simulink model "TrajectoryControl_Team"  (R2022b)
settings: Solver=FixedStepAuto  StartTime=0.0  StopTime=30  FixedStep=0.001  RelTol=1e-3
undefined symbols (not defined in the file): h, headingAngle, km, m, Moment_limit, s, smiData, Steering_Angle, Vehicle_Speed, x, X, Y, Z
libraries: sm_lib x213, aerolibconvert2 x17, simulink_extras x14, nesl_utility x14, spsMosfetLib x4, autolibshared x3, slpidlib x2, eePwmGenerator x1, spsDCVoltageSourceLib x1, spsVoltageMeasurementLib x1, sps_lib x1, autolibutils x1
(part 1 of 6)
settings Model: Creator=dangm  LastModifiedBy=Lenovo
settings SolverCC: ZeroCrossAlgorithm=Adaptive  AlgebraicLoopSolver=LineSearch
settings DebuggingCC: IgnoredZcDiagnostic=none  UnconnectedInputMsg=warning  UnconnectedOutputMsg=warning  UnconnectedLineMsg=warning  SFMachineParentedDataDiag=warning
settings ModelReferenceCC: EnableRefExpFcnMdlSchedulingChecks=on
settings ExplorerConfigSet: InternalSimMechanicsExplorerSettings="<ExplorerConfiguration><canonicalview>planar_xy</canonicalview><AnimationSetting><BasePlaybackSpeed>1.0</BasePlaybackSpeed><PlaybackSpeedFactor>1.0</PlaybackSpeedFactor></AnimationSetting><TilePanel><TileInfo><Tiles Columns=\"1\" Count=\"1\" Rows=\"1\"><Column Weight=\"1\"/><Row Weight=\"1\"/><Tile Height=\"1\" Width=\"1\" X=\"0\" Y=\"0\"/></Tiles></TileInfo><SceneInfo><SceneViewer><BGColor><R>0.60000002384185791</R><G>0.60000002384185791</G><B>0.60000002384185791</B></BGColor><Camera><DoPerspective>off</DoPerspective><Position><X>1.38151927744802361</X><Y>-0.113937833645223696</Y><Z>-0.183681847979671575</Z></Position><Center><X>0.0576620377884289326</X><Y>0.060665039066758325</Y><Z>0.733764197719871003</Z></Center><Up><X>0.27535581417737931</X><Y>0.936019488942585909</Y><Z>0.219195556338108416</Z></Up><ViewLimDist>1</ViewLimDist><YLim>0.747285369634628327</YLim><XLim>1.35610315607225207</XLim></Camera></SceneViewer></SceneInfo></TilePanel><MechEditorPanel><Cameras/><GfxPanelCameraMap/><VideoCreator><PlaybackSpeedRatio>1.0</PlaybackSpeedRatio><FrameRate>30</FrameRate><VideoFormat>Motion JPEG AVI</VideoFormat><FrameSize>auto</FrameSize></VideoCreator></MechEditorPanel></ExplorerConfiguration>"

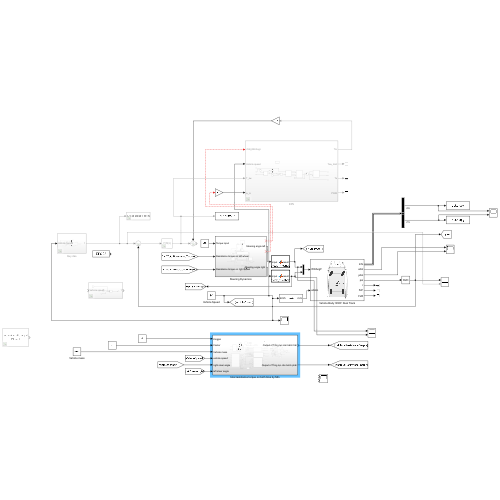
[thumbnail: Simulink's stored preview of the top-level diagram]
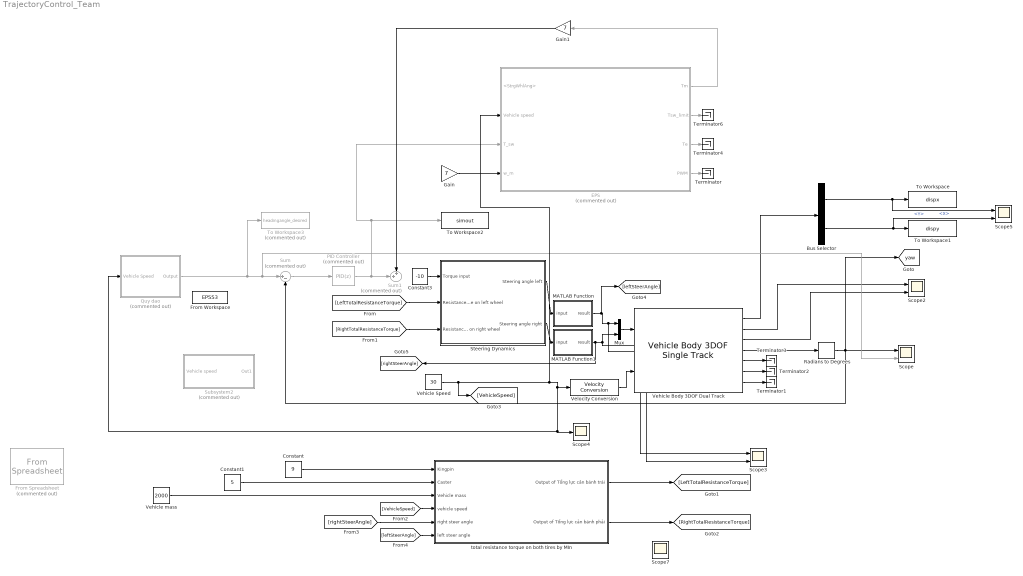
== system TrajectoryControl_Team ==
  Bus Selector : BusSelector  OutputSignals=InertFrm.Cg.Disp.X,InertFrm.Cg.Disp.Y
  Constant : Constant  Value=9
  Constant1 : Constant  Value=5
  Constant3 : Constant  Value=-10
  EPS : Subsystem  Commented=on
  From Workspace : FromWorkspace  VariableName=EPSS3
  From Spreadsheet : FromSpreadsheet  Commented=on  FileName=Khao sat khoi luong.xlsx  Range=A3:B13
  Gain : Gain  Gain=7
  Gain1 : Gain  Gain=7
  MATLAB Function : MATLAB Function  TreatAsAtomicUnit=on
  MATLAB Function1 : MATLAB Function  TreatAsAtomicUnit=on
  Mux : Mux  Inputs=2
  PID Controller : slpidlib/PID Controller  Commented=on  Controller=PID  Form=Parallel  TimeDomain=Discrete-time  UseExternalTs=off  SampleTime=-1  IntegratorMethod=Forward Euler  FilterMethod=Forward Euler  ControllerParametersSource=internal  P=1  I=0  UseKiTs=off  D=20  N=205.123568338568  UseFilter=off  TunerSelectOption=Transfer Function Based (PID Tuner App)  InitialConditionSource=internal  InitialConditionForIntegrator=0  InitialConditionForFilter=0  DifferentiatorICPrevScaledInput=0  ExternalReset=none  TrackingMode=off  Kt=1  LimitOutput=off  SatLimitsSource=internal  UpperSaturationLimit=0  LowerSaturationLimit=-10  LinearizeAsGain=on  AntiWindupMode=none  Kb=1  LimitIntegrator=off  UpperIntegratorSaturationLimit=inf  LowerIntegratorSaturationLimit=-inf  POutMin=[]  POutMax=[]  IOutMin=[]  IOutMax=[]  DOutMin=[]  DOutMax=[]  NOutMin=[]  NOutMax=[]  SumOutMin=[]  SumOutMax=[]  SaturationOutMin=[]  SaturationOutMax=[]  PParamMin=[]  PParamMax=[]  IParamMin=[]  IParamMax=[]  DParamMin=[]  DParamMax=[]  NParamMin=[]  NParamMax=[]  KbParamMin=[]  KbParamMax=[]  KtParamMin=[]  KtParamMax=[]  KbOutMin=[]  KbOutMax=[]  KtOutMin=[]  KtOutMax=[]  IntegratorOutMin=[]  IntegratorOutMax=[]  FilterOutMin=[]  FilterOutMax=[]  SumI1OutMin=[]  SumI1OutMax=[]  SumI2OutMin=[]  SumI2OutMax=[]  SumI3OutMin=[]  SumI3OutMax=[]  SumI4OutMin=[]  SumI4OutMax=[]  SumDOutMin=[]  SumDOutMax=[]  DifferentiatorOutMin=[]  DifferentiatorOutMax=[]  FilterDiffOutCoefMin=[]  FilterDiffOutCoefMax=[]  ReciprocalOutMin=[]  ReciprocalOutMax=[]  SumDenOutMin=[]  SumDenOutMax=[]  SumNumOutMin=[]  SumNumOutMax=[]  DivideOutMin=[]  DivideOutMax=[]  UdiffTsProdOutMin=[]  UdiffTsProdOutMax=[]  NTsProdOutMin=[]  NTsProdOutMax=[]  UintegralTsProdOutMin=[]  UintegralTsProdOutMax=[]  UngainTsProdOutMin=[]  UngainTsProdOutMax=[]  ClampingZeroOutDataTypeStr=Inherit: Inherit via back propagation  ClampingZeroOutMin=[]  ClampingZeroOutMax=[]  FilterDenConstantOutDataTypeStr=Inherit: Inherit via back propagation  FilterDenConstantOutMin=[]  FilterDenConstantOutMax=[]  PCopyOutDataTypeStr=Inherit: Inherit via back propagation  PCopyOutMin=[]  PCopyOutMax=[]  NCopyOutDataTypeStr=Inherit: Inherit via back propagation  NCopyOutMin=[]  NCopyOutMax=[]  IntegratorContinuousStateAttributes=''  IntegratorStateMustResolveToSignalObject=off  IntegratorRTWStateStorageClass=Auto  FilterContinuousStateAttributes=''  FilterStateMustResolveToSignalObject=off  FilterRTWStateStorageClass=Auto  ParallelPVariant=InternalParameters  IdealPVariant=Disabled  IVariant=InternalParameters  DVariant=InternalParameters  IntegratorVariant=Discrete  SatVariant=Disabled  AWVariant=Passthrough  PCopyVariant=Disabled  TRVariant=Disabled  FdbkBlocksVariant=Forward  IdealPFdbkVariant=Disabled  SatFdbkVariant=Disabled  DerivativeFilterVariant=Differentiator  NVariant=Passthrough  NCopyVariant=Disabled_SignalSpec  FilterICVariant=InternalICsDifferentiator  IntegratorICVariant=InternalICs  ExternalResetVariant=Disabled  TRSumVariant=Passthrough  SumFdbkVariant=Disabled  SumVariant=Sum_PID  TsampFilterVariant=InternalTs  TsampNgainVariant=Passthrough  TsampIntegralVariant=Passthrough  ExternalSaturationOutDataTypeStr=Inherit: Same as second input
  Quy dao : Subsystem  Commented=on
  Radians to Degrees : simulink_extras/Transformations/Radians to Degrees
  Scope{,2..3,5,7} (5 alike) : Scope  NumInputPorts=2
  Scope4 : Scope
  Steering Dynamics : Subsystem
  Subsystem2 : Subsystem  Commented=on
  Sum : Sum  Commented=on  Inputs=|+-
  Sum1 : Sum  Commented=on  Inputs=++|
  Terminator{,1..4,6} (6 alike) : Terminator
  To Workspace : ToWorkspace  VariableName=dispx  SaveFormat=Structure With Time  SampleTime=-1
  To Workspace1 : ToWorkspace  VariableName=dispy  SaveFormat=Structure With Time  SampleTime=-1
  To Workspace2 : ToWorkspace  VariableName=simout  SaveFormat=Structure With Time  SampleTime=-1
  To Workspace3 : ToWorkspace  Commented=on  VariableName=headingangle_desired  SaveFormat=Structure With Time  SampleTime=-1
  Vehicle Body 3DOF Dual Track : autolibshared/Vehicle Body 3DOF Single Track  trackMode=Dual  inputMode=External longitudinal velocity  frontSteerMode=on  rearSteerMode=off  windMode=off  muMode=off  extFMode=off  extMMode=off  htchFMode=off  htchMMode=off  extXo=off  extpsio=off  extxdoto=off  extro=off  extYo=off  extTamb=off  extydoto=off  aMode=2  NF=2  NR=2  m=2000  a=1.4  b=1.6  h=0.35  dh=1  hh=0.2  X_o=0  xdot_o=0  CalphaMode=off  sigmaMode=on  d=0  hl=0  w=[1.4,1.4]  Cy_f=12e3  Cy_r=11e3  sigma_f=.1  sigma_r=.1  alpha_f_brk=[-.1 .1]  Cy_f_data=[-9e3 9e3]  alpha_r_brk=[-.1 .1]  Cy_r_data=[-9e3 9e3]  Y_o=0  ydot_o=0  Izz=4000  psi_o=0  r_o=0  Af=2  Cd=.3  Cl=.1  Cpm=.1  beta_w=[0:0.01:0.3]  Cs=[0:0.03:0.9]  Cym=[0:0.01:0.3]  Pabs=101325  Tair=273  g=9.81  mu=1  xdot_tol=.01  Fznom=5000  Fxtire_sat=7e4  Fytire_sat=7e4  longOff=0  latOff=0  vertOff=0  wrapAng=off
  Vehicle Speed : Constant  Value=30
  Vehicle mass : Constant  Value=2000
  Velocity Conversion : aerolibconvert2/Velocity Conversion  IU=km/h  OU=m/s
  total resistance torque on both tires by MIn : Subsystem
  tag scope: yaw=global
  wires:
  Mux/1 -> Vehicle Body 3DOF Dual Track/1
  Vehicle Body 3DOF Dual Track/6 -> Terminator2/1
  Vehicle Body 3DOF Dual Track/5 -> Terminator3/1
  Vehicle Body 3DOF Dual Track/1 -> Bus Selector/1
  Vehicle Body 3DOF Dual Track/3 -> Scope2/2
  Vehicle Body 3DOF Dual Track/4 -> Radians to Degrees/1
  Radians to Degrees/1 -> [yaw], Scope/1, Sum/2
  Bus Selector/1 -> Scope5/1, To Workspace/1  "<X>"
  Bus Selector/2 -> Scope5/2, To Workspace1/1  "<Y>"
  Velocity Conversion/1 -> Vehicle Body 3DOF Dual Track/2
  Vehicle Body 3DOF Dual Track/2 -> Scope2/1
  Sum/1 -> PID Controller/1
  Quy dao/1(Output) -> To Workspace3/1, Scope/2, Sum/1
  ? -> EPS/1(<StrgWhlAng>)
  ? -> Gain/1
  Steering Dynamics/1(Steering angle left) -> MATLAB Function/1(input)
  Steering Dynamics/2(Steering angle right) -> MATLAB Function1/1(input)
  MATLAB Function1/1(result) -> [rightSteerAngle], Mux/2, Scope3/2
  PID Controller/1 -> Sum1/2, EPS/3(T_sw), To Workspace2/1
  Constant/1 -> total resistance torque on both tires by MIn/1(Kingpin)
  Constant1/1 -> total resistance torque on both tires by MIn/2(Caster)
  Vehicle mass/1 -> total resistance torque on both tires by MIn/3(Vehicle mass)
  Gain/1 -> EPS/4(w_m)
  EPS/4(PWM) -> Terminator/1
  EPS/3(Te) -> Terminator4/1
  EPS/2(Tsw_limit) -> Terminator6/1
  EPS/1(Tm) -> Gain1/1
  Gain1/1 -> Sum1/1
  Vehicle Speed/1 -> EPS/2(Vehicle speed), Quy dao/1("Vehicle Speed "), Scope4/1, Velocity Conversion/1, [VehicleSpeed]
  MATLAB Function/1(result) -> [leftSteerAngle], Scope3/1, Mux/1
  Constant3/1 -> Steering Dynamics/1(Torque input)
  total resistance torque on both tires by MIn/1(Output of Tổng lực cản bánh trái) -> [LeftTotalResistanceTorque]
  total resistance torque on both tires by MIn/2(Output of Tổng lực cản bánh phải) -> [RightTotalResistanceTorque]
  [LeftTotalResistanceTorque] -> Steering Dynamics/2(Resistance torque on left wheel)
  [RightTotalResistanceTorque] -> Steering Dynamics/3(Resistance torque on right wheel)
  [VehicleSpeed] -> total resistance torque on both tires by MIn/4("vehicle speed ")
  [rightSteerAngle] -> total resistance torque on both tires by MIn/5(right steer angle)
  [leftSteerAngle] -> total resistance torque on both tires by MIn/6(left steer angle)
  Vehicle Body 3DOF Dual Track/7 -> Terminator1/1

== system TrajectoryControl_Team/EPS ==
  <StrgWhlAng> : Inport
  Vehicle speed : Inport  Port=2
  T_sw : Inport  Port=3
  w_m : Inport  Port=4
  Abs : Abs  SaturateOnIntegerOverflow=off
  Abs2 : Abs  SaturateOnIntegerOverflow=off
  Constant : Constant  Value=0
  Lookup_Table : Subsystem
  Moment Controller : Subsystem
  Motor 1 : Subsystem  mask{Km=0.456, Kb=0.3533, B=0.071, J=0.00218907, L=0.002, R=0.6}
      mask prompts: Km "Torque constant"; Kb "Back emf constant"; B "Viscous friction"; J "Inertia"; L "Inductance"; R "Resistance"
      mask Display: image('motor.png');
  Motor Driver : Subsystem
      mask Display: image('bridge.png');
  Sum2 : Sum  Inputs=+|-||
  Switch : Switch  Criteria=u2 > Threshold  SaturateOnIntegerOverflow=off  InputSameDT=off
  Va : spsVoltageMeasurementLib/Voltage Measurement  Tag=PoWeRsYsTeMmEaSuReMeNt  PhasorSimulation=off  OutputType=Magnitude  PSBequivalent=0
  powergui : sps_lib/powergui  Priority=1  SimulationMode=Discrete  SampleTime=0.00001  frequency=60  Iterations=50  frequencyindice=0  Pbase=100e6  ErrMax=1e-4  UnitsV=kV  UnitsW=MW  buscounter=0  FunctionMessages=off  echomessages=off  EnableUseOfTLC=off  CurrentSourceSwitches=off  DisableSnubberDevices=off  DisableRonSwitches=off  DisableVfSwitches=off  DisplayEquations=off  AutomaticDiscreteSolvers=off  SolverType=Tustin/Backward Euler (TBE)  Interpol=off  ExternalGateDelay=off  methode=off  Ts=100  x0status=blocks  SPID=on  SwTol=0  HookPort=off  NonlinearTolerance=1e-4  nMaxIteration=100  ContinueOnMaxIteration=off  RestoreLinks=warning  ResistiveCurrentMeasurement=off  Frange=[0:2:500]  Ylog=off  Xlog=on  ShowGrid=off  save=off  variable=ZData  structure=0  ZoomFFT=off  StartTime=0.0  cycles=1  DisplayStyle=1  fundamental=60  FreqAxis=off  MaxFrequency=1000  frequencyindicesteady=1  RmsSteady=1  display=off
  Tm : Outport  VectorParamsAs1DForOutWhenUnconnected=off
  Tsw_limit : Outport  Port=2  VectorParamsAs1DForOutWhenUnconnected=off
  Te : Outport  Port=3  VectorParamsAs1DForOutWhenUnconnected=off
  PWM : Outport  Port=4  VectorParamsAs1DForOutWhenUnconnected=off
  wires:
  Abs2/1 -> Lookup_Table/1(theta_sw)
  Moment Controller/1(PWM1) -> Motor Driver/1(PWM1)
  Moment Controller/4(PWM4) -> Motor Driver/4(PWM4)
  Switch/1 -> Moment Controller/2(error)
  T_sw/1 -> Moment Controller/1(Direction), Abs/1
  Moment Controller/2(PWM2) -> Motor Driver/2(PWM2)
  <StrgWhlAng>/1 -> Abs2/1
  Moment Controller/3(PWM3) -> Motor Driver/3(PWM3)
  w_m/1 -> Motor 1/2(wm)
  Va/1 -> Motor 1/1(U), PWM/1
  Sum2/1 -> Switch/2, Switch/1  "e_Tsw"
  Constant/1 -> Switch/3
  Abs/1 -> Sum2/1
  Motor 1/2(Te) -> Te/1
  Motor 1/1(Tm) -> Tm/1
  Vehicle speed/1 -> Lookup_Table/2(vc)
  Lookup_Table/1(Tsw_limit) -> Sum2/2, Tsw_limit/1  "Tsw_limit"
  connections:
  Motor Driver/LConn1 -- Va/LConn2
  Motor Driver/RConn1 -- Va/LConn1

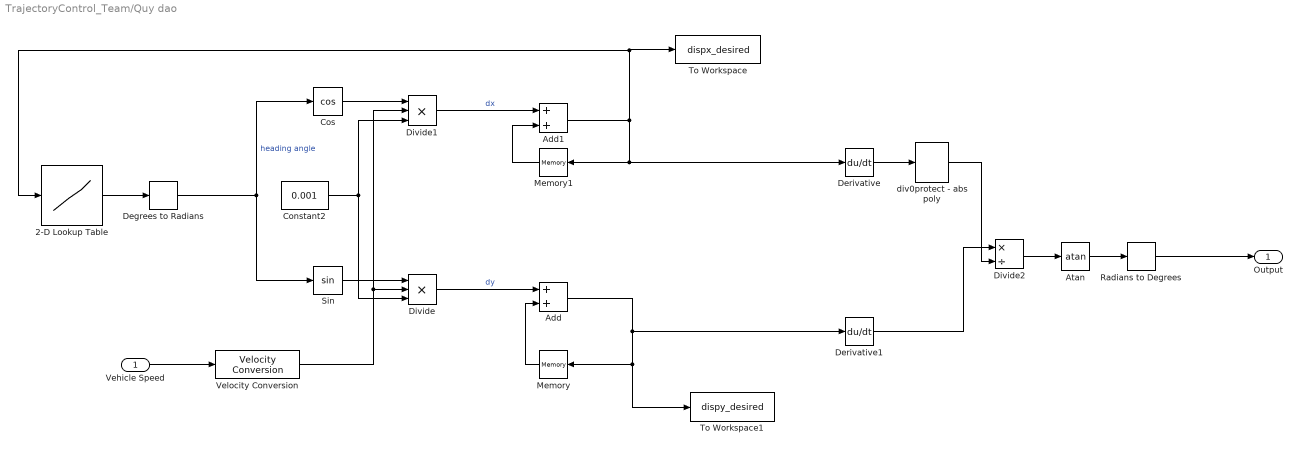
== system TrajectoryControl_Team/Quy dao ==
  "Vehicle Speed " : Inport
  2-D Lookup Table : Lookup_n-D  NumberOfTableDimensions=1  BreakpointsForDimension1=x  BreakpointsForDimension2=[1:3]  Table=headingAngle  InternalRulePriority=Speed  RndMeth=Simplest
  Add : Sum
  Add1 : Sum
  Atan : Trigonometry  Operator=atan
  Constant2 : Constant  Value=0.001
  Cos : Trigonometry  Operator=cos
  Degrees to Radians : simulink_extras/Transformations/Degrees to Radians
  Derivative : Derivative
  Derivative1 : Derivative
  Divide : Product  Inputs=***
  Divide1 : Product  Inputs=***
  Divide2 : Product  Inputs=*/
  Memory : Memory
  Memory1 : Memory
  Radians to Degrees : simulink_extras/Transformations/Radians to Degrees
  Sin : Trigonometry
  To Workspace : ToWorkspace  VariableName=dispx_desired  SaveFormat=Structure With Time  SampleTime=-1
  To Workspace1 : ToWorkspace  VariableName=dispy_desired  SaveFormat=Structure With Time  SampleTime=-1
  Velocity Conversion : aerolibconvert2/Velocity Conversion  IU=km/h  OU=m/s
  div0protect - abs poly : autolibutils/div0protect - abs poly  thresh=1e-6  aMode=aMode
  Output : Outport
  wires:
  Constant2/1 -> Divide/3, Divide1/3
  Sin/1 -> Divide/1
  Degrees to Radians/1 -> Sin/1, Cos/1  "heading angle"
  Atan/1 -> Radians to Degrees/1
  Add/1 -> Memory/1, To Workspace1/1, Derivative1/1
  "Vehicle Speed "/1 -> Velocity Conversion/1
  Velocity Conversion/1 -> Divide/2, Divide1/2
  Divide1/1 -> Add1/1  "dx"
  Derivative/1 -> div0protect - abs poly/1
  Memory/1 -> Add/2
  Add1/1 -> Memory1/1, Derivative/1, 2-D Lookup Table/1, To Workspace/1
  Cos/1 -> Divide1/1
  Derivative1/1 -> Divide2/1
  Divide2/1 -> Atan/1
  Divide/1 -> Add/1  "dy"
  Memory1/1 -> Add1/2
  2-D Lookup Table/1 -> Degrees to Radians/1
  div0protect - abs poly/1 -> Divide2/2
  Radians to Degrees/1 -> Output/1

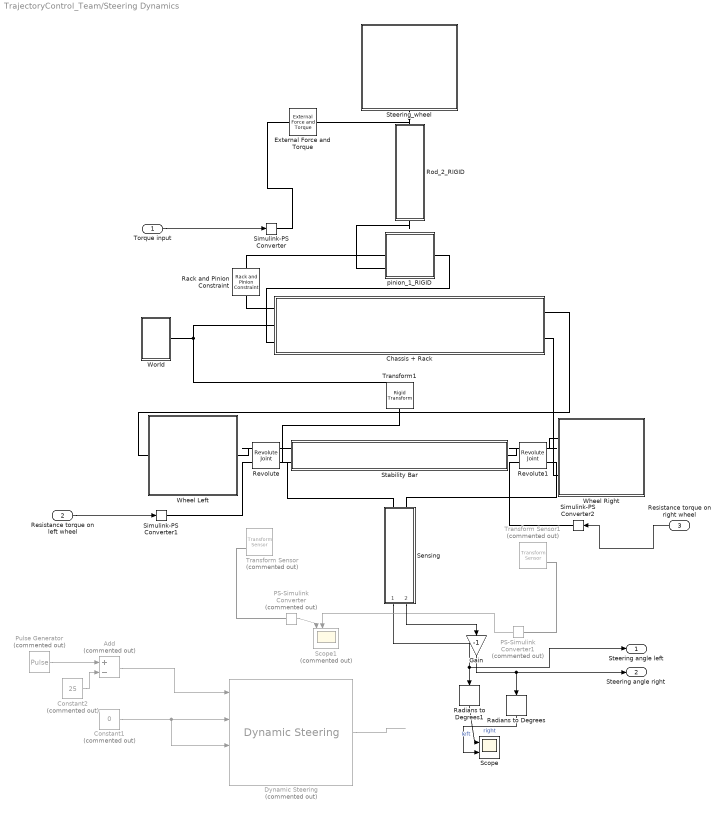
== system TrajectoryControl_Team/Steering Dynamics ==
  Torque input : Inport
  Resistance torque on left wheel : Inport  Port=2
  Resistance torque on right wheel : Inport  Port=3
  Add : Sum  Commented=on  Inputs=+-
  Chassis + Rack : Subsystem
  Constant1 : Constant  Commented=on  Value=0
  Constant2 : Constant  Commented=on  Value=25
  Dynamic Steering : vehdynlibsteering/Dynamic Steering  Commented=on  StrgType=Rack and pinion  StrgRatioType=Constant  PwrAst=off  Loc=Front  TrckWdth=1  WhlBase=1.524  StrgRng=1.25*pi  StrgAngBpts="[-6.2832   -5.0265   -3.7699   -2.5133   -1.2566         0    1.2566    2.5133    3.7699    5.0265    6.2832]"  StrgRatioTbl=|  StrgRatio=13.5  StrgArmLngth=0.1  RckCsLngth=0.5  TieRodLngth=0.248  D=0.2  PnnRadiusTbl="[0.0055    0.0055    0.0056    0.0057    0.0057    0.0057    0.0058    0.0057    0.0056    0.0055    0.0055]"  PnnRadius=0.0057  RodLngth=0.1  ParaArmLngth=0.9  J1=0.1  J2=0.01  beta_u=0.1  beta_l=0.1  b1=0.001  k1=30  b2=1  b3=0.001  theta_o=0  omega_o=0  FricTrq=0  TrqBpts=[-100 0 100]  VehSpdBpts=[0 20]  TrqTbl=[0 -100;0 0;0 100]  TrqLmt=100  PwrLmt=1000  Eta=1  omega_c=200  aMode=2
      | [13.5000   13.3750   13.2500   13.1250   13.0000   13.0000   13.0000   13.1250   13.2500   13.3750   13.5000
      | ]
  External Force and Torque : sm_lib/Forces and Torques/External Force and Torque  ForceResolutionFrame=AttachedFrame  EnableForceX=off  EnableForceY=off  EnableForceZ=off  EnableForce=off  TorqueResolutionFrame=AttachedFrame  EnableTorqueX=off  EnableTorqueY=off  EnableTorqueZ=on  EnableTorque=off
  Gain : Gain  Gain=-1
  PS-Simulink Converter : nesl_utility/PS-Simulink Converter  Commented=on  PhysicalDomain=network_engine_domain  SubClassName=ps_output  LeftPortType=input  RightPortType=output  PseudoPeriodic=off  Frequencies=[]  VectorFormat=1-D array  Unit=inherit  AffineConversion=off
  PS-Simulink Converter1 : nesl_utility/PS-Simulink Converter  Commented=on  PhysicalDomain=network_engine_domain  SubClassName=ps_output  LeftPortType=input  RightPortType=output  PseudoPeriodic=off  Frequencies=[]  VectorFormat=1-D array  Unit=inherit  AffineConversion=off
  Pulse Generator : DiscretePulseGenerator  Commented=on  PulseType=Time based  Amplitude=50  Period=10  PulseWidth=50
  Rack and Pinion Constraint : sm_lib/Gears and Couplings/Gears/Rack and Pinion Constraint  PinionRadius=30  PinionRadiusUnits=mm
  Radians to Degrees : simulink_extras/Transformations/Radians to Degrees
  Radians to Degrees1 : simulink_extras/Transformations/Radians to Degrees
  Revolute : sm_lib/Joints/Revolute Joint  JointMode=Normal  SenseConstraintForce=off  SenseConstraintForceX=off  SenseConstraintForceY=off  SenseConstraintForceZ=off  SenseConstraintTorque=off  SenseConstraintTorqueX=off  SenseConstraintTorqueY=off  SenseConstraintTorqueZ=off  SenseTotalForce=off  SenseTotalForceX=off  SenseTotalForceY=off  SenseTotalForceZ=off  SenseTotalTorque=off  SenseTotalTorqueX=off  SenseTotalTorqueY=off  SenseTotalTorqueZ=off  CompositeWrenchDir=FollowerOnBase  CompositeWrenchFrame=BaseFrame  EquilibriumPosition=0  EquilibriumPositionUnits=deg  SpringStiffness=0.0524  SpringStiffnessUnits=N*m/deg  DampingCoefficient=1.5  DampingCoefficientUnits=N*m/(deg/s)  TorqueActuationMode=InputTorque  MotionActuationMode=ComputedMotion  SensePosition=on  SenseVelocity=off  SenseAcceleration=off  SenseTorqueForce=off  SenseLowerLimitTorqueForce=off  SenseUpperLimitTorqueForce=off  LowerLimitSpecify=on  LowerLimitBound=-2  LowerLimitBoundUnits=rad  LowerLimitStiffness=1e4  LowerLimitStiffnessUnits=N*m/deg  LowerLimitDamping=100  LowerLimitDampingUnits=N*m/(deg/s)  LowerLimitTransitionRegionWidth=0.1  LowerLimitTransitionRegionWidthUnits=deg  UpperLimitSpecify=on  UpperLimitBound=-1  UpperLimitBoundUnits=rad  UpperLimitStiffness=1e4  UpperLimitStiffnessUnits=N*m/deg  UpperLimitDamping=100  UpperLimitDampingUnits=N*m/(deg/s)  UpperLimitTransitionRegionWidth=0.1  UpperLimitTransitionRegionWidthUnits=deg  PositionTargetSpecify=on  PositionTargetPriority=High  PositionTargetValue=-89.678329494  PositionTargetValueUnits=deg  VelocityTargetSpecify=on  VelocityTargetPriority=High  VelocityTargetValue=0  VelocityTargetValueUnits=deg/s
  Revolute1 : sm_lib/Joints/Revolute Joint  JointMode=Normal  SenseConstraintForce=off  SenseConstraintForceX=off  SenseConstraintForceY=off  SenseConstraintForceZ=off  SenseConstraintTorque=off  SenseConstraintTorqueX=off  SenseConstraintTorqueY=off  SenseConstraintTorqueZ=off  SenseTotalForce=off  SenseTotalForceX=off  SenseTotalForceY=off  SenseTotalForceZ=off  SenseTotalTorque=off  SenseTotalTorqueX=off  SenseTotalTorqueY=off  SenseTotalTorqueZ=off  CompositeWrenchDir=FollowerOnBase  CompositeWrenchFrame=BaseFrame  EquilibriumPosition=0  EquilibriumPositionUnits=deg  SpringStiffness=0.0524  SpringStiffnessUnits=N*m/deg  DampingCoefficient=1.5  DampingCoefficientUnits=N*m/(deg/s)  TorqueActuationMode=InputTorque  MotionActuationMode=ComputedMotion  SensePosition=on  SenseVelocity=off  SenseAcceleration=off  SenseTorqueForce=off  SenseLowerLimitTorqueForce=off  SenseUpperLimitTorqueForce=off  LowerLimitSpecify=on  LowerLimitBound=-2  LowerLimitBoundUnits=rad  LowerLimitStiffness=1e4  LowerLimitStiffnessUnits=N*m/deg  LowerLimitDamping=100  LowerLimitDampingUnits=N*m/(deg/s)  LowerLimitTransitionRegionWidth=0.1  LowerLimitTransitionRegionWidthUnits=deg  UpperLimitSpecify=on  UpperLimitBound=-1  UpperLimitBoundUnits=rad  UpperLimitStiffness=1e4  UpperLimitStiffnessUnits=N*m/deg  UpperLimitDamping=100  UpperLimitDampingUnits=N*m/(deg/s)  UpperLimitTransitionRegionWidth=0.1  UpperLimitTransitionRegionWidthUnits=deg  PositionTargetSpecify=on  PositionTargetPriority=Low  PositionTargetValue=smiData.RevoluteJoint(2).Rz.Pos-2.7  PositionTargetValueUnits=deg  VelocityTargetSpecify=on  VelocityTargetPriority=High  VelocityTargetValue=0  VelocityTargetValueUnits=deg/s
  Rod_2_RIGID : Subsystem
      mask Display: image('rod.png'); % Use "Edit Image" on toolstrip to change.
  Scope : Scope  NumInputPorts=2
  Scope1 : Scope  Commented=on  NumInputPorts=4
  "Sensing " : Subsystem
  Simulink-PS Converter : nesl_utility/Simulink-PS Converter  PhysicalDomain=network_engine_domain  SubClassName=ps_input  LeftPortType=input  RightPortType=output  PseudoPeriodic=off  Frequencies=[]  NoiseDistribution=none  NoiseParameters=[]  Unit=N*m  AffineConversion=off  FilteringAndDerivatives=provide  SimscapeFilterOrder=1  InputFilterTimeConstant=0.001  UdotUserProvided=0
  Simulink-PS Converter1 : nesl_utility/Simulink-PS Converter  PhysicalDomain=network_engine_domain  SubClassName=ps_input  LeftPortType=input  RightPortType=output  PseudoPeriodic=off  Frequencies=[]  NoiseDistribution=none  NoiseParameters=[]  Unit=N*m  AffineConversion=off  FilteringAndDerivatives=provide  SimscapeFilterOrder=1  InputFilterTimeConstant=0.001  UdotUserProvided=0
  Simulink-PS Converter2 : nesl_utility/Simulink-PS Converter  PhysicalDomain=network_engine_domain  SubClassName=ps_input  LeftPortType=input  RightPortType=output  PseudoPeriodic=off  Frequencies=[]  NoiseDistribution=none  NoiseParameters=[]  Unit=N*m  AffineConversion=off  FilteringAndDerivatives=provide  SimscapeFilterOrder=2  InputFilterTimeConstant=0.001  UdotUserProvided=0
  Stability Bar : Subsystem
      mask Display: image('E:\Hoc\do an\(final) download\test14\image\stability bar.png'); % Use "Edit Image" on toolstrip to change.
  Steering_wheel : Subsystem
      mask Display: image('$imagefile'); % Use "Edit Image" on toolstrip to change.
  Transform Sensor : sm_lib/Frames and Transforms/Transform Sensor  Commented=on  MeasurementFrame=Base  SenseAngle=on  SenseAxis=off  SenseQ=off  SenseR=off  SenseRotationSequence=off  RotationSequence=XYX  SenseOmegaX=off  SenseOmegaY=off  SenseOmegaZ=off  SenseQDot=off  SenseRDot=off  SenseAlphaX=off  SenseAlphaY=off  SenseAlphaZ=off  SenseQDDot=off  SenseRDDot=off  SenseX=off  SenseY=off  SenseZ=off  SenseRad=off  SenseAzim=off  SenseDist=off  SenseInc=off  SenseXDot=off  SenseYDot=off  SenseZDot=off  SenseRadDot=off  SenseAzimDot=off  SenseDistDot=off  SenseIncDot=off  SenseXDDot=off  SenseYDDot=off  SenseZDDot=off  SenseRadDDot=off  SenseAzimDDot=off  SenseDistDDot=off  SenseIncDDot=off
  Transform Sensor1 : sm_lib/Frames and Transforms/Transform Sensor  Commented=on  MeasurementFrame=Base  SenseAngle=on  SenseAxis=off  SenseQ=off  SenseR=off  SenseRotationSequence=off  RotationSequence=XYX  SenseOmegaX=off  SenseOmegaY=off  SenseOmegaZ=off  SenseQDot=off  SenseRDot=off  SenseAlphaX=off  SenseAlphaY=off  SenseAlphaZ=off  SenseQDDot=off  SenseRDDot=off  SenseX=off  SenseY=off  SenseZ=off  SenseRad=off  SenseAzim=off  SenseDist=off  SenseInc=off  SenseXDot=off  SenseYDot=off  SenseZDot=off  SenseRadDot=off  SenseAzimDot=off  SenseDistDot=off  SenseIncDot=off  SenseXDDot=off  SenseYDDot=off  SenseZDDot=off  SenseRadDDot=off  SenseAzimDDot=off  SenseDistDDot=off  SenseIncDDot=off
  Transform1 : sm_lib/Frames and Transforms/Rigid Transform  TranslationMethod=Cartesian  TranslationStandardOffset=0  TranslationLengthUnit=mm  TranslationStandardAxis=+Z  TranslationCartesianOffset=smiData.RigidTransform(48).translation  TranslationROffset=0  TranslationROffsetUnits=m  TranslationZOffset=0  TranslationZOffsetUnits=m  TranslationThetaOffset=0  TranslationThetaOffsetUnits=deg  RotationMethod=ArbitraryAxis  RotationAngleUnits=rad  RotationStandardAxis=+Z  RotationAngle=smiData.RigidTransform(48).angle  RotationArbitraryAxis=smiData.RigidTransform(48).axis  FollAlignAxisA=+X  BaseAlignAxisA=+Y  FollAlignAxisB=+Y  BaseAlignAxisB=+Z  RotationSequenceAxes=FollowerAxes  RotationSequence=XYX  RotationSequenceAngles=[0 0 0]  RotationSequenceAnglesUnits=deg  RotationMatrix=[1 0 0; 0 1 0; 0 0 1]  Quaternion=[1 0 0 0]
  Wheel Left : Subsystem
      mask Display: image('E:\Hoc\do an\(final) download\test14\image\wheel.png'); % Use "Edit Image" on toolstrip to change.
  Wheel Right : Subsystem
      mask Display: image('E:\Hoc\do an\(final) download\test14\image\wheel.png'); % Use "Edit Image" on toolstrip to change.
  World : Subsystem
  pinion_1_RIGID : Subsystem
      mask Display: image('pinion.png'); % Use "Edit Image" on toolstrip to change.
  Steering angle left : Outport
  Steering angle right : Outport  Port=2
  wires:
  "Sensing "/1(Steering angle left (rad)) -> Steering angle left/1, Radians to Degrees1/1
  Add/1 -> Dynamic Steering/1
  Pulse Generator/1 -> Add/1
  Gain/1 -> Steering angle right/1, Radians to Degrees/1
  PS-Simulink Converter1/1 -> Scope1/2
  Constant2/1 -> Add/2
  Constant1/1 -> Dynamic Steering/3, Dynamic Steering/2
  Dynamic Steering/2 -> ?
  "Sensing "/2(Steering angle right (rad)) -> Gain/1
  PS-Simulink Converter/1 -> Scope1/1
  Torque input/1 -> Simulink-PS Converter/1
  Radians to Degrees/1 -> Scope/2  "right"
  Radians to Degrees1/1 -> Scope/1  "left"
  Resistance torque on left wheel/1 -> Simulink-PS Converter1/1
  Resistance torque on right wheel/1 -> Simulink-PS Converter2/1
  connections:
  PS-Simulink Converter1/LConn1 -- Transform Sensor1/RConn2
  Revolute/RConn2 -- "Sensing "/LConn1
  Simulink-PS Converter/RConn1 -- External Force and Torque/LConn1
  Chassis + Rack/LConn2 -- World/LConn1 -- Transform1/LConn1
  Rack and Pinion Constraint/RConn1 -- Chassis + Rack/LConn1
  PS-Simulink Converter/LConn1 -- Transform Sensor/RConn2
  "Sensing "/LConn2 -- Revolute1/RConn2
  Rack and Pinion Constraint/LConn1 -- pinion_1_RIGID/LConn2
  Transform1/RConn1 -- Stability Bar/LConn2
  Chassis + Rack/LConn3 -- pinion_1_RIGID/RConn1
  Chassis + Rack/RConn1 -- Wheel Left/LConn1
  Revolute1/RConn1 -- Wheel Right/LConn1
  Chassis + Rack/RConn2 -- Wheel Right/LConn2
  Revolute1/LConn1 -- Stability Bar/RConn1
  Revolute/RConn1 -- Stability Bar/LConn1
  Revolute/LConn1 -- Wheel Left/RConn1
  Rod_2_RIGID/RConn1 -- pinion_1_RIGID/LConn3
  Steering_wheel/LConn1 -- External Force and Torque/RConn1 -- Rod_2_RIGID/LConn1
  Simulink-PS Converter1/RConn1 -- Revolute/LConn2
  Simulink-PS Converter2/RConn1 -- Revolute1/LConn2

== system TrajectoryControl_Team/Subsystem2 ==
  Vehicle speed : Inport
  Constant : Constant  Value=10
  Switch : Switch  Criteria=u2 > Threshold  SaturateOnIntegerOverflow=off  InputSameDT=off
  Out1 : Outport
  wires:
  Switch/1 -> Out1/1
  [yaw] -> Switch/2
  Constant/1 -> Switch/1
  Vehicle speed/1 -> Switch/3

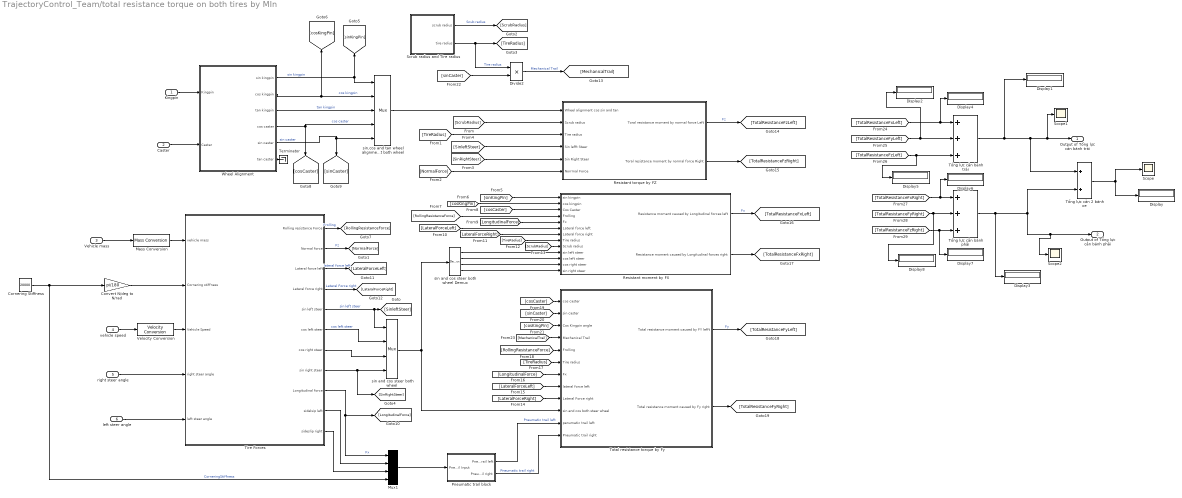
== system TrajectoryControl_Team/total resistance torque on both tires by MIn ==
  Kingpin : Inport
  Caster : Inport  Port=2
  Vehicle mass : Inport  Port=3
  "vehicle speed " : Inport  Port=4
  right steer angle : Inport  Port=5
  left steer angle : Inport  Port=6
  Convert N/deg to N/rad : Gain  Gain=pi/180
  Cornering Stiffness : Constant  Value=20000
  Display{,1..8} (9 alike) : Display
  Divide2 : Product  Inputs=**
  Mass Conversion : aerolibconvert2/Mass Conversion  IU=kg  OU=kg
  Mux1 : Mux
  Pneumatic trail block : Subsystem
  Resistant moment by FX : Subsystem
  Resistant torque by FZ : Subsystem
  Scope : Scope
  Scope1 : Scope
  Scope2 : Scope
  Scrub radius and Tire radius : Subsystem
  Terminator : Terminator
  Tire Forces : Subsystem
  Total resistance torque by Fy : Subsystem
  Tổng lực cản 2 bánh xe : Sum
  Tổng lực cản bánh phải : Sum  Inputs=+++
  Tổng lực cản bánh trái : Sum  Inputs=+++
  Velocity Conversion : aerolibconvert2/Velocity Conversion  IU=km/h  OU=m/s
  Wheel Alignment : Subsystem
  sin and cos steer both wheel : Mux
  sin and cos steer both wheel Demux : Demux
  sin,cos and tan wheel alignment both wheel : Mux  Inputs=5
  Output of Tổng lực cản bánh trái : Outport
  Output of Tổng lực cản bánh phải : Outport  Port=2
  wires:
  Kingpin/1 -> Wheel Alignment/1(Kingpin)
  Wheel Alignment/6(tan caster) -> Terminator/1
  Vehicle mass/1 -> Mass Conversion/1
  Mass Conversion/1 -> Tire Forces/1(vehicle mass)
  Convert N/deg to N/rad/1 -> Tire Forces/2(Cornering stiffness)
  Cornering Stiffness/1 -> Mux1/4, Convert N/deg to N/rad/1  "CorneringStiffness"
  Caster/1 -> Wheel Alignment/2(Caster)
  "vehicle speed "/1 -> Velocity Conversion/1
  right steer angle/1 -> Tire Forces/4("right steer angle ")
  left steer angle/1 -> Tire Forces/5("left steer angle ")
  Velocity Conversion/1 -> Tire Forces/3(Vehicle Speed)
  Tire Forces/11(sideslip right) -> Mux1/3
  Tire Forces/10(sidelsip left) -> Mux1/2
  Tire Forces/9(Longitudinal force) -> [LongitudinalForce], Mux1/1  "Fx"
  Mux1/1 -> Pneumatic trail block/1(Pneumatic trail Input)
  Pneumatic trail block/2(Pneumatic Trail right) -> Total resistance torque by Fy/12(Pneumatic trail right)  "Pneumatic trail right"
  Pneumatic trail block/1(Pneumatic Trail left) -> Total resistance torque by Fy/11(penumatic trail left)  "Pneumatic trail left"
  Tire Forces/5(sin left steer) -> sin and cos steer both wheel/1, [SinleftSteer]  "sin left steer"
  Tire Forces/6(cos left steer) -> sin and cos steer both wheel/2  "cos left steer"
  Tire Forces/7(cos right steer) -> sin and cos steer both wheel/3
  Tire Forces/8(sin right steer) -> [SinRightSteer], sin and cos steer both wheel/4
  sin and cos steer both wheel/1 -> sin and cos steer both wheel Demux/1, Total resistance torque by Fy/10(sin and cos both steer wheel)
  Wheel Alignment/1(sin kingpin) -> sin,cos and tan wheel alignment both wheel/1, [sinKingPin]  "sin kingpin"
  Wheel Alignment/2(cos kingpin) -> [cosKingPin], sin,cos and tan wheel alignment both wheel/2  "cos kingpin"
  Wheel Alignment/3(tan kingpin) -> sin,cos and tan wheel alignment both wheel/3  "tan kingpin"
  Wheel Alignment/4(cos caster) -> sin,cos and tan wheel alignment both wheel/4, [cosCaster]  "cos caster"
  Wheel Alignment/5(sin caster) -> [sinCaster], sin,cos and tan wheel alignment both wheel/5  "sin caster"
  sin,cos and tan wheel alignment both wheel/1 -> Resistant torque by FZ/1("Wheel alignment cos sin and tan ")
  Tire Forces/2(Normal force) -> [NormalForce]  "Fz"
  Scrub radius and Tire radius/1(scrub radius) -> [ScrubRadius]  "Scub radius"
  Scrub radius and Tire radius/2(tire radius) -> Divide2/1, [TireRadius]  "Tire radius"
  [ScrubRadius] -> Resistant torque by FZ/2(Scrub radius)
  [TireRadius] -> Resistant torque by FZ/3(Tire radius)
  [NormalForce] -> Resistant torque by FZ/6(Norrmal Force)
  [SinleftSteer] -> Resistant torque by FZ/4(Sin lefft Steer)
  [SinRightSteer] -> Resistant torque by FZ/5(Sin Right Steer)
  [sinKingPin] -> Resistant moment by FX/1(sin kingpin)
  [cosKingPin] -> Resistant moment by FX/2(cos kingpin)
  Tire Forces/1(Rolling resistance Force) -> [RollingResistanceForce]  "Frolling"
  [RollingResistanceForce] -> Resistant moment by FX/4(Frolling)
  [cosCaster] -> Resistant moment by FX/3(Cos Caster)
  [LongitudinalForce] -> Resistant moment by FX/5(Fx)
  Tire Forces/3(Lateral force left) -> [LateralForceLeft]  "lateral force left"
  Tire Forces/4(Lateral force right) -> [LateralForceRight]  "Lateral Force right"
  [LateralForceLeft] -> Resistant moment by FX/6(Lateral force left)
  [LateralForceRight] -> Resistant moment by FX/7(Lateral force right)
  [TireRadius] -> Resistant moment by FX/8(Tire radius)
  [ScrubRadius] -> Resistant moment by FX/9(Scrub radius)
  [LateralForceRight] -> Total resistance torque by Fy/9(Lateral Force right)
  [LateralForceLeft] -> Total resistance torque by Fy/8(lateral force left)
  [LongitudinalForce] -> Total resistance torque by Fy/7(Fx)
  [TireRadius] -> Total resistance torque by Fy/6(Tire radius)
  [RollingResistanceForce] -> Total resistance torque by Fy/5(Frolling)
  [sinCaster] -> Total resistance torque by Fy/2(sin caster)
  [cosCaster] -> Total resistance torque by Fy/1(cos caster)
  [cosKingPin] -> Total resistance torque by Fy/3(Cos Kingpin angle)
  sin and cos steer both wheel Demux/1 -> Resistant moment by FX/10(sin left steer)
  sin and cos steer both wheel Demux/2 -> Resistant moment by FX/11(cos left steer)
  sin and cos steer both wheel Demux/3 -> Resistant moment by FX/12(cos right steer)
  sin and cos steer both wheel Demux/4 -> Resistant moment by FX/13(sin right steer)
  [sinCaster] -> Divide2/2
  Divide2/1 -> [MechanicalTrail]  "Mechanical Trail"
  [MechanicalTrail] -> Total resistance torque by Fy/4(Mechanical Trail)
  Resistant torque by FZ/1(Toral resistance moment by normal force Left) -> [TotalResistanceFzLeft]  "Fz"
  Resistant torque by FZ/2(Toral resistance moment by normal force Right) -> [TotalResistanceFzRight]
  Resistant moment by FX/1(Resistance moment caused by Longitudinal forces left) -> [TotalResistanceFxLeft]  "Fx"
  Resistant moment by FX/2(Resistance moment caused by Longitudinal forces right) -> [TotalResistanceFxRight]
  Total resistance torque by Fy/2(Total resistance moment caused by Fy right) -> [TotalResistanceFyRight]
  Total resistance torque by Fy/1("Total resistance moment caused by FY lefft ") -> [TotalResistanceFyLeft]  "Fy"
  [TotalResistanceFxLeft] -> Tổng lực cản bánh trái/1, Display4/1
  [TotalResistanceFyLeft] -> Display2/1, Tổng lực cản bánh trái/2
  [TotalResistanceFzLeft] -> Display5/1, Tổng lực cản bánh trái/3
  [TotalResistanceFxRight] -> Display6/1, Tổng lực cản bánh phải/1
  [TotalResistanceFyRight] -> Display8/1, Tổng lực cản bánh phải/2
  [TotalResistanceFzRight] -> Display7/1, Tổng lực cản bánh phải/3
  Tổng lực cản bánh trái/1 -> Display1/1, Scope1/1, Output of Tổng lực cản bánh trái/1, Tổng lực cản 2 bánh xe/1
  Tổng lực cản bánh phải/1 -> Display3/1, Scope2/1, Output of Tổng lực cản bánh phải/1, Tổng lực cản 2 bánh xe/2
  Tổng lực cản 2 bánh xe/1 -> Scope/1, Display/1

== system TrajectoryControl_Team/EPS/Lookup_Table ==
  theta_sw : Inport
      mask Display: image('1.png');
  vc : Inport  Port=2
      mask Display: image('speed.png');
  2-D Lookup Table : Lookup_n-D  BreakpointsForDimension1=Steering_Angle  BreakpointsForDimension2=Vehicle_Speed  Table=Moment_limit  InternalRulePriority=Speed  RndMeth=Simplest
      settings: InputPortMap=u0,u1
  Tsw_limit : Outport  VectorParamsAs1DForOutWhenUnconnected=off
  wires:
  theta_sw/1 -> 2-D Lookup Table/1
  vc/1 -> 2-D Lookup Table/2
  2-D Lookup Table/1 -> Tsw_limit/1

== system TrajectoryControl_Team/EPS/Moment Controller ==
  Direction : Inport
  error : Inport  Port=2
  Abs : Abs  ZeroCross=off  SaturateOnIntegerOverflow=off
  Constant{,1..3} (4 alike) : Constant  Value=0
  Controller : Subsystem
  Demux1 : Demux
  Mux : Mux
  Mux1 : Mux
  PWM Generator : eePwmGenerator/PWM Generator  CarrCount=Up  Tper=0.0001  Tdelay=0  Ts=0.00001
  Saturation : Saturate  UpperLimit=1  LowerLimit=0
  Scope : Scope
  Switch : Switch  SaturateOnIntegerOverflow=off  InputSameDT=off
  PWM1 : Outport  VectorParamsAs1DForOutWhenUnconnected=off
  PWM2 : Outport  Port=2  VectorParamsAs1DForOutWhenUnconnected=off
  PWM3 : Outport  Port=3  VectorParamsAs1DForOutWhenUnconnected=off
  PWM4 : Outport  Port=4  VectorParamsAs1DForOutWhenUnconnected=off
  wires:
  Demux1/1 -> PWM1/1
  Demux1/4 -> PWM4/1
  Demux1/3 -> PWM3/1
  Demux1/2 -> PWM2/1
  Mux1/1 -> Switch/1
  Mux/1 -> Switch/3
  Switch/1 -> Demux1/1
  Constant2/1 -> Mux1/2
  Constant3/1 -> Mux1/3
  Constant/1 -> Mux/1
  Constant1/1 -> Mux/4
  Controller/1(duty_cycle) -> Saturation/1
  PWM Generator/1 -> Scope/1, Mux/2, Mux/3, Mux1/1, Mux1/4
  Saturation/1 -> PWM Generator/1
  Abs/1 -> Controller/1(error)
  error/1 -> Abs/1
  Direction/1 -> Switch/2

== system TrajectoryControl_Team/EPS/Motor 1 ==
  U : Inport
  wm : Inport  Port=2
  1/L : Fcn  Expr=u/L
  Abs : Abs  SaturateOnIntegerOverflow=off
  Constant : Constant  Value=0
  Derivative : Derivative
  Gain : Gain  Gain=Km
  Gain1 : Gain  Gain=B
  Gain2 : Gain  Gain=R
  Gain3 : Gain  Gain=Kb
  Gain5 : Gain  Gain=J
  Integrator : Integrator
  Sum : Sum  Inputs=|-+-|
  Sum1 : Sum  Inputs=|+--
  Switch : Switch  Criteria=u2 > Threshold  SaturateOnIntegerOverflow=off  InputSameDT=off
  Tm : Outport  VectorParamsAs1DForOutWhenUnconnected=off
  Te : Outport  Port=2  VectorParamsAs1DForOutWhenUnconnected=off
  wires:
  Sum/1 -> 1/L/1
  1/L/1 -> Integrator/1  "di/dt"
  Integrator/1 -> Gain2/1, Gain/1  "i"
  Gain/1 -> Te/1, Sum1/1  "Te"
  Gain2/1 -> Sum/1  "i.R"
  Gain1/1 -> Sum1/2  "Tf"
  Sum1/1 -> Tm/1
  Derivative/1 -> Gain5/1
  Gain5/1 -> Sum1/3  "Tj"
  wm/1 -> Derivative/1, Gain1/1, Gain3/1
  U/1 -> Abs/1, Sum/2
  Abs/1 -> Switch/2
  Gain3/1 -> Switch/1  "Kb.w_m"
  Constant/1 -> Switch/3
  Switch/1 -> Sum/3

== system TrajectoryControl_Team/EPS/Motor Driver ==
  PWM1 : Inport
  PWM2 : Inport  Port=2
  PWM3 : Inport  Port=3
  PWM4 : Inport  Port=4
  DC Voltage Source : spsDCVoltageSourceLib/DC Voltage Source  Amplitude=36  Measurements=Voltage
  Mosfet{1..4} (4 alike) : spsMosfetLib/Mosfet  Ron=0.1  Lon=0  Rd=0.01  Vfd=0  IC=0  Rs=1e5  Cs=inf  Measurements=on
  Terminator{,1..3} (4 alike) : Terminator
  + : PMIOPort  Side=Right
  - : PMIOPort  Port=2  Side=Left
  wires:
  PWM3/1 -> Mosfet3/1
  PWM1/1 -> Mosfet1/1
  PWM2/1 -> Mosfet2/1
  PWM4/1 -> Mosfet4/1
  Mosfet1/1 -> Terminator/1
  Mosfet3/1 -> Terminator1/1
  Mosfet2/1 -> Terminator2/1
  Mosfet4/1 -> Terminator3/1
  connections:
  Mosfet4/RConn1 -- DC Voltage Source/LConn1 -- Mosfet2/RConn1
  Mosfet2/LConn1 -- Mosfet1/RConn1 -- +/RConn1
  Mosfet3/LConn1 -- DC Voltage Source/RConn1 -- Mosfet1/LConn1
  Mosfet3/RConn1 -- -/RConn1 -- Mosfet4/LConn1

== system TrajectoryControl_Team/Steering Dynamics/Chassis + Rack ==
  Rack Case + Chassis : Subsystem
  Rack_1_RIGID : Subsystem
  Target : PMIOPort  Side=Left
  Conn3 : PMIOPort  Port=2  Side=Left
  Conn1 : PMIOPort  Port=3  Side=Left
  F2 : PMIOPort  Port=4  Side=Right
  F3 : PMIOPort  Port=5  Side=Right
  connections:
  Rack_1_RIGID/RConn1 -- Rack Case + Chassis/LConn2
  Rack_1_RIGID/RConn2 -- Rack Case + Chassis/LConn3
  Rack_1_RIGID/RConn4 -- Rack Case + Chassis/LConn5
  Conn3/RConn1 -- Rack Case + Chassis/LConn1
  Target/RConn1 -- Rack_1_RIGID/LConn1
  Rack Case + Chassis/LConn4 -- Rack_1_RIGID/RConn3
  Rack Case + Chassis/LConn7 -- F2/RConn1
  Rack Case + Chassis/LConn6 -- Rack_1_RIGID/RConn5
  Rack Case + Chassis/RConn2 -- F3/RConn1
  Rack Case + Chassis/RConn1 -- Conn1/RConn1

== system TrajectoryControl_Team/Steering Dynamics/Rod_2_RIGID ==
  ReferenceFrame : sm_lib/Frames and Transforms/Reference Frame
  Solid : sm_lib/Body Elements/File Solid  ExtGeomFileName=Rod_Default_sldprt.STEP  UnitType=FromFile  ExtGeomFileUnits=m  StepReaderType=HEX  ExportConvexHullGeometry=off  InertiaType=Custom  Mass=smiData.Solid(4).mass  MassUnits=kg  CenterOfMass=smiData.Solid(4).CoM  CenterOfMassUnits=mm  MomentsOfInertia=smiData.Solid(4).MoI  MomentsOfInertiaUnits=kg*mm^2  ProductsOfInertia=smiData.Solid(4).PoI  ProductsOfInertiaUnits=kg*mm^2  BasedOnType=DensityFromFile  Density=1000  DensityUnits=kg/m^3  DoExposeReferenceFrame=on  SerializedFrames=<Frames/>  GraphicType=FromGeometry  MarkerShape=Sphere  MarkerSize=10  GraphicVisPropType=SimpleVisualProperties  GraphicDiffuseColor=smiData.Solid(4).color  GraphicSpecularColor=[0.5 0.5 0.5 1.0]  GraphicAmbientColor=[0.15 0.15 0.15 1.0]  GraphicEmissiveColor=[0.0 0.0 0.0 1.0]  GraphicShininess=75  GraphicOpacity=smiData.Solid(4).opacity
  Transform : sm_lib/Frames and Transforms/Rigid Transform  TranslationMethod=Cartesian  TranslationStandardOffset=0  TranslationLengthUnit=mm  TranslationStandardAxis=+Z  TranslationCartesianOffset=smiData.RigidTransform(39).translation  TranslationROffset=0  TranslationROffsetUnits=m  TranslationZOffset=0  TranslationZOffsetUnits=m  TranslationThetaOffset=0  TranslationThetaOffsetUnits=deg  RotationMethod=ArbitraryAxis  RotationAngleUnits=rad  RotationStandardAxis=+Z  RotationAngle=smiData.RigidTransform(39).angle  RotationArbitraryAxis=smiData.RigidTransform(39).axis  FollAlignAxisA=+X  BaseAlignAxisA=+Y  FollAlignAxisB=+Y  BaseAlignAxisB=+Z  RotationSequenceAxes=FollowerAxes  RotationSequence=XYX  RotationSequenceAngles=[0 0 0]  RotationSequenceAnglesUnits=deg  RotationMatrix=[1 0 0; 0 1 0; 0 0 1]  Quaternion=[1 0 0 0]
  Transform1 : sm_lib/Frames and Transforms/Rigid Transform  TranslationMethod=Cartesian  TranslationStandardOffset=0  TranslationLengthUnit=mm  TranslationStandardAxis=+Z  TranslationCartesianOffset=smiData.RigidTransform(42).translation  TranslationROffset=0  TranslationROffsetUnits=m  TranslationZOffset=0  TranslationZOffsetUnits=m  TranslationThetaOffset=0  TranslationThetaOffsetUnits=deg  RotationMethod=ArbitraryAxis  RotationAngleUnits=rad  RotationStandardAxis=+Z  RotationAngle=smiData.RigidTransform(42).angle  RotationArbitraryAxis=smiData.RigidTransform(42).axis  FollAlignAxisA=+X  BaseAlignAxisA=+Y  FollAlignAxisB=+Y  BaseAlignAxisB=+Z  RotationSequenceAxes=FollowerAxes  RotationSequence=XYX  RotationSequenceAngles=[0 0 0]  RotationSequenceAnglesUnits=deg  RotationMatrix=[1 0 0; 0 1 0; 0 0 1]  Quaternion=[1 0 0 0]
  F : PMIOPort  Side=Left
  F1 : PMIOPort  Port=2  Side=Right
  connections:
  Solid/RConn1 -- ReferenceFrame/RConn1 -- Transform/LConn1 -- Transform1/LConn1
  Transform/RConn1 -- F/RConn1
  Transform1/RConn1 -- F1/RConn1

== system TrajectoryControl_Team/Steering Dynamics/Sensing  ==
  Add : Sum
  Add1 : Sum
  Constant1 : Constant  Value=1.5458-2.6414e-05+0.01940853136
  Constant2 : Constant  Value=1.5847-(-2.3866e-05)-0.019541748665
  PS-Simulink Converter : nesl_utility/PS-Simulink Converter  PhysicalDomain=network_engine_domain  SubClassName=ps_output  LeftPortType=input  RightPortType=output  PseudoPeriodic=off  Frequencies=[]  VectorFormat=1-D array  Unit=rad  AffineConversion=off
  PS-Simulink Converter1 : nesl_utility/PS-Simulink Converter  PhysicalDomain=network_engine_domain  SubClassName=ps_output  LeftPortType=input  RightPortType=output  PseudoPeriodic=off  Frequencies=[]  VectorFormat=1-D array  Unit=rad  AffineConversion=off
  Radians to Degrees : simulink_extras/Transformations/Radians to Degrees
  Radians to Degrees1 : simulink_extras/Transformations/Radians to Degrees
  Scope : Scope  NumInputPorts=2
  To Workspace : ToWorkspace  VariableName=left  SaveFormat=Structure  SampleTime=-1
  To Workspace1 : ToWorkspace  VariableName=right  SaveFormat=Structure  SampleTime=-1
  input : PMIOPort  Side=Left
  input1 : PMIOPort  Port=2  Side=Left
  Steering angle left (rad) : Outport
  Steering angle right (rad) : Outport  Port=2
  wires:
  Constant1/1 -> Add/2
  PS-Simulink Converter1/1 -> Radians to Degrees1/1, Add1/1, To Workspace1/1  "Steering angle right (rad)"
  PS-Simulink Converter/1 -> To Workspace/1, Radians to Degrees/1, Add/1  "Steering angle left (rad)"
  Constant2/1 -> Add1/2
  Add/1 -> Steering angle left (rad)/1  "Steering angle left (rad)"
  Add1/1 -> Steering angle right (rad)/1  "Steering angle right (rad)"
  Radians to Degrees/1 -> Scope/1  "left"
  Radians to Degrees1/1 -> Scope/2  "right"
  connections:
  input/RConn1 -- PS-Simulink Converter/LConn1
  input1/RConn1 -- PS-Simulink Converter1/LConn1

== system TrajectoryControl_Team/Steering Dynamics/Stability Bar ==
  ReferenceFrame : sm_lib/Frames and Transforms/Reference Frame
  Solid : sm_lib/Body Elements/File Solid  ExtGeomFileName=lock_arm by Long_Default_sldprt.STEP  UnitType=FromFile  ExtGeomFileUnits=m  StepReaderType=HEX  ExportConvexHullGeometry=off  InertiaType=Custom  Mass=smiData.Solid(12).mass  MassUnits=kg  CenterOfMass=smiData.Solid(12).CoM  CenterOfMassUnits=mm  MomentsOfInertia=smiData.Solid(12).MoI  MomentsOfInertiaUnits=kg*mm^2  ProductsOfInertia=smiData.Solid(12).PoI  ProductsOfInertiaUnits=kg*mm^2  BasedOnType=DensityFromFile  Density=1000  DensityUnits=kg/m^3  DoExposeReferenceFrame=on  SerializedFrames=<Frames/>  GraphicType=FromGeometry  MarkerShape=Sphere  MarkerSize=10  GraphicVisPropType=SimpleVisualProperties  GraphicDiffuseColor=smiData.Solid(12).color  GraphicSpecularColor=[0.5 0.5 0.5 1.0]  GraphicAmbientColor=[0.15 0.15 0.15 1.0]  GraphicEmissiveColor=[0.0 0.0 0.0 1.0]  GraphicShininess=75  GraphicOpacity=smiData.Solid(12).opacity
  Transform : sm_lib/Frames and Transforms/Rigid Transform  TranslationMethod=Cartesian  TranslationStandardOffset=0  TranslationLengthUnit=mm  TranslationStandardAxis=+Z  TranslationCartesianOffset=smiData.RigidTransform(2).translation  TranslationROffset=0  TranslationROffsetUnits=m  TranslationZOffset=0  TranslationZOffsetUnits=m  TranslationThetaOffset=0  TranslationThetaOffsetUnits=deg  RotationMethod=ArbitraryAxis  RotationAngleUnits=rad  RotationStandardAxis=+Z  RotationAngle=smiData.RigidTransform(2).angle  RotationArbitraryAxis=smiData.RigidTransform(2).axis  FollAlignAxisA=+X  BaseAlignAxisA=+Y  FollAlignAxisB=+Y  BaseAlignAxisB=+Z  RotationSequenceAxes=FollowerAxes  RotationSequence=XYX  RotationSequenceAngles=[0 0 0]  RotationSequenceAnglesUnits=deg  RotationMatrix=[1 0 0; 0 1 0; 0 0 1]  Quaternion=[1 0 0 0]
  Transform1 : sm_lib/Frames and Transforms/Rigid Transform  TranslationMethod=Cartesian  TranslationStandardOffset=0  TranslationLengthUnit=mm  TranslationStandardAxis=+Z  TranslationCartesianOffset=smiData.RigidTransform(3).translation  TranslationROffset=0  TranslationROffsetUnits=m  TranslationZOffset=0  TranslationZOffsetUnits=m  TranslationThetaOffset=0  TranslationThetaOffsetUnits=deg  RotationMethod=ArbitraryAxis  RotationAngleUnits=rad  RotationStandardAxis=+Z  RotationAngle=smiData.RigidTransform(3).angle  RotationArbitraryAxis=smiData.RigidTransform(3).axis  FollAlignAxisA=+X  BaseAlignAxisA=+Y  FollAlignAxisB=+Y  BaseAlignAxisB=+Z  RotationSequenceAxes=FollowerAxes  RotationSequence=XYX  RotationSequenceAngles=[0 0 0]  RotationSequenceAnglesUnits=deg  RotationMatrix=[1 0 0; 0 1 0; 0 0 1]  Quaternion=[1 0 0 0]
  F : PMIOPort  Side=Left
  F2 : PMIOPort  Port=2  Side=Left
  F1 : PMIOPort  Port=3  Side=Right
  connections:
  Solid/RConn1 -- ReferenceFrame/RConn1 -- Transform/LConn1 -- Transform1/LConn1 -- F2/RConn1
  Transform/RConn1 -- F/RConn1
  Transform1/RConn1 -- F1/RConn1

== system TrajectoryControl_Team/Steering Dynamics/Steering_wheel ==
  ReferenceFrame : sm_lib/Frames and Transforms/Reference Frame
  Solid : sm_lib/Body Elements/File Solid  ExtGeomFileName=Steering wheel_Default_sldprt.STEP  UnitType=FromFile  ExtGeomFileUnits=m  StepReaderType=HEX  ExportConvexHullGeometry=off  InertiaType=Custom  Mass=smiData.Solid(9).mass  MassUnits=kg  CenterOfMass=smiData.Solid(9).CoM  CenterOfMassUnits=mm  MomentsOfInertia=smiData.Solid(9).MoI  MomentsOfInertiaUnits=kg*mm^2  ProductsOfInertia=smiData.Solid(9).PoI  ProductsOfInertiaUnits=kg*mm^2  BasedOnType=DensityFromFile  Density=1000  DensityUnits=kg/m^3  DoExposeReferenceFrame=on  SerializedFrames=<Frames/>  GraphicType=FromGeometry  MarkerShape=Sphere  MarkerSize=10  GraphicVisPropType=SimpleVisualProperties  GraphicDiffuseColor=smiData.Solid(9).color  GraphicSpecularColor=[0.5 0.5 0.5 1.0]  GraphicAmbientColor=[0.15 0.15 0.15 1.0]  GraphicEmissiveColor=[0.0 0.0 0.0 1.0]  GraphicShininess=75  GraphicOpacity=smiData.Solid(9).opacity
  Transform : sm_lib/Frames and Transforms/Rigid Transform  TranslationMethod=Cartesian  TranslationStandardOffset=0  TranslationLengthUnit=mm  TranslationStandardAxis=+Z  TranslationCartesianOffset=smiData.RigidTransform(40).translation  TranslationROffset=0  TranslationROffsetUnits=m  TranslationZOffset=0  TranslationZOffsetUnits=m  TranslationThetaOffset=0  TranslationThetaOffsetUnits=deg  RotationMethod=ArbitraryAxis  RotationAngleUnits=rad  RotationStandardAxis=+Z  RotationAngle=smiData.RigidTransform(40).angle  RotationArbitraryAxis=smiData.RigidTransform(40).axis  FollAlignAxisA=+X  BaseAlignAxisA=+Y  FollAlignAxisB=+Y  BaseAlignAxisB=+Z  RotationSequenceAxes=FollowerAxes  RotationSequence=XYX  RotationSequenceAngles=[0 0 0]  RotationSequenceAnglesUnits=deg  RotationMatrix=[1 0 0; 0 1 0; 0 0 1]  Quaternion=[1 0 0 0]
  F : PMIOPort  Side=Left
  connections:
  Solid/RConn1 -- ReferenceFrame/RConn1 -- Transform/LConn1
  Transform/RConn1 -- F/RConn1

== system TrajectoryControl_Team/Steering Dynamics/Wheel Left ==
  Innova_Crysta_Assembly_Final_1_RIGID : Subsystem
  wheelpin_by_Long_1_RIGID : Subsystem
  F2 : PMIOPort  Side=Left
  F : PMIOPort  Port=2  Side=Right
  connections:
  Innova_Crysta_Assembly_Final_1_RIGID/RConn1 -- wheelpin_by_Long_1_RIGID/LConn1
  F2/RConn1 -- wheelpin_by_Long_1_RIGID/RConn2
  F/RConn1 -- wheelpin_by_Long_1_RIGID/RConn1

== system TrajectoryControl_Team/Steering Dynamics/Wheel Right ==
  Innova_Crysta_Assembly_Final_2_RIGID : Subsystem
  wheelpin_by_Long_2_RIGID : Subsystem
  F : PMIOPort  Side=Left
  F2 : PMIOPort  Port=2  Side=Left
  connections:
  Innova_Crysta_Assembly_Final_2_RIGID/RConn1 -- wheelpin_by_Long_2_RIGID/RConn1
  F2/RConn1 -- wheelpin_by_Long_2_RIGID/LConn2
  F/RConn1 -- wheelpin_by_Long_2_RIGID/LConn1
